simulink model "c00002M_harness"  (R2018a)
settings: Solver=FixedStepAuto  StartTime=0.0  StopTime=300  FixedStep=0.1  RelTol=1e-3
undefined symbols (not defined in the file): A1, hmax, R1, R2, sigbuilder_block, TempThreshold
(part 1 of 14)
settings Model: Creator=aarrieta  LastModifiedBy=umarkiegi

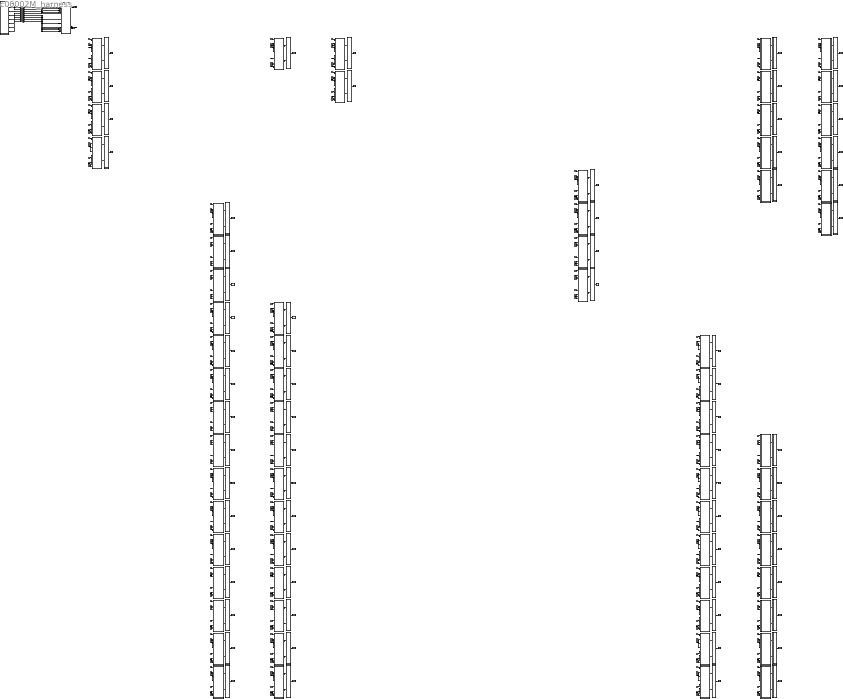
== system c00002M_harness ==
  CPSUT : Subsystem
  Eval : Subsystem
  Eval1 : Subsystem
  Eval164 : Subsystem
  Eval165 : Subsystem
  Eval166 : Subsystem
  Eval167 : Subsystem
  Eval2 : Subsystem
  Eval209 : Subsystem
  Eval210 : Subsystem
  Eval211 : Subsystem
  Eval212 : Subsystem
  Eval213 : Subsystem
  Eval214 : Subsystem
  Eval215 : Subsystem
  Eval216 : Subsystem
  Eval217 : Subsystem
  Eval218 : Subsystem
  Eval219 : Subsystem
  Eval220 : Subsystem
  Eval221 : Subsystem
  Eval222 : Subsystem
  Eval223 : Subsystem
  Eval224 : Subsystem
  Eval232 : Subsystem
  Eval233 : Subsystem
  Eval234 : Subsystem
  Eval235 : Subsystem
  Eval236 : Subsystem
  Eval237 : Subsystem
  Eval238 : Subsystem
  Eval239 : Subsystem
  Eval240 : Subsystem
  Eval241 : Subsystem
  Eval242 : Subsystem
  Eval243 : Subsystem
  Eval244 : Subsystem
  Eval245 : Subsystem
  Eval3 : Subsystem
  Eval45 : Subsystem
  Eval46 : Subsystem
  Eval47 : Subsystem
  Eval48 : Subsystem
  Eval49 : Subsystem
  Eval50 : Subsystem
  Eval51 : Subsystem
  Eval52 : Subsystem
  Eval53 : Subsystem
  Eval54 : Subsystem
  Eval55 : Subsystem
  Eval56 : Subsystem
  Eval57 : Subsystem
  Eval58 : Subsystem
  Eval59 : Subsystem
  Eval60 : Subsystem
  Eval68 : Subsystem
  Eval69 : Subsystem
  Eval70 : Subsystem
  Eval71 : Subsystem
  Eval72 : Subsystem
  Eval73 : Subsystem
  Eval74 : Subsystem
  Eval75 : Subsystem
  Eval76 : Subsystem
  Eval77 : Subsystem
  Eval78 : Subsystem
  Eval79 : Subsystem
  Eval80 : Subsystem
  Eval81 : Subsystem
  Inputs : Subsystem  Tag=STV Subsys  LoadFcn=sigbuilder_block('load');  StartFcn=sigbuilder_block('start');  StopFcn=sigbuilder_block('stop');  ClipboardFcn=sigbuilder_block('clipboard');  mask(Sigbuilder block){tuvar=[0:10]}
      mask init:
      | if ~strcmp(get_param(bdroot(gcb),'SimulationStatus'),'stopped'),tuvar = sigbuilder_block('maskInit'); end
      settings: CopyFcn=sigbuilder_block('copy');  DeleteFcn=sigbuilder_block('delete');  ModelCloseFcn=sigbuilder_block('modelClose');  PreSaveFcn=sigbuilder_block('preSave');  PauseFcn=sigbuilder_block('pause');  ContinueFcn=sigbuilder_block('continue');  NameChangeFcn=sigbuilder_block('namechange');  OpenFcn=sigbuilder_block('open',[276.75 163.5 675.75 486.75 ]);  CloseFcn=sigbuilder_block('close');
      mask Display: plot(0, 0, 100, 100,[2, 2, 32, 32, 2], [68, 8, 8, 68, 68],[32, 2], [38, 38], [32, 19, 2],[53, 60, 44], [32, 17, 17, 2],[16, 16, 31, 31]);txt = getActiveGroup(gcbh);text(2, 100, txt,'verticalAlignment', 'top');
  M001 : Subsystem
  M002 : Subsystem
  M003 : Subsystem
  M004 : Subsystem
  M046 : Subsystem
  M047 : Subsystem
  M048 : Subsystem
  M049 : Subsystem
  M050 : Subsystem
  M051 : Subsystem
  M052 : Subsystem
  M053 : Subsystem
  M054 : Subsystem
  M055 : Subsystem
  M056 : Subsystem
  M057 : Subsystem
  M058 : Subsystem
  M059 : Subsystem
  M060 : Subsystem
  M061 : Subsystem
  M069 : Subsystem
  M070 : Subsystem
  M071 : Subsystem
  M072 : Subsystem
  M073 : Subsystem
  M074 : Subsystem
  M075 : Subsystem
  M076 : Subsystem
  M077 : Subsystem
  M078 : Subsystem
  M079 : Subsystem
  M080 : Subsystem
  M081 : Subsystem
  M082 : Subsystem
  M165 : Subsystem
  M166 : Subsystem
  M167 : Subsystem
  M168 : Subsystem
  M210 : Subsystem
  M211 : Subsystem
  M212 : Subsystem
  M213 : Subsystem
  M214 : Subsystem
  M215 : Subsystem
  M216 : Subsystem
  M217 : Subsystem
  M218 : Subsystem
  M219 : Subsystem
  M220 : Subsystem
  M221 : Subsystem
  M222 : Subsystem
  M223 : Subsystem
  M224 : Subsystem
  M225 : Subsystem
  M233 : Subsystem
  M234 : Subsystem
  M235 : Subsystem
  M236 : Subsystem
  M237 : Subsystem
  M238 : Subsystem
  M239 : Subsystem
  M240 : Subsystem
  M241 : Subsystem
  M242 : Subsystem
  M243 : Subsystem
  M244 : Subsystem
  M245 : Subsystem
  M246 : Subsystem
  To Workspace : ToWorkspace  VariableName=mutant001  SampleTime=-1
  To Workspace1 : ToWorkspace  VariableName=mutant002  SampleTime=-1
  To Workspace164 : ToWorkspace  VariableName=mutant165  SampleTime=-1
  To Workspace165 : ToWorkspace  VariableName=mutant166  SampleTime=-1
  To Workspace166 : ToWorkspace  VariableName=mutant167  SampleTime=-1
  To Workspace167 : ToWorkspace  VariableName=mutant168  SampleTime=-1
  To Workspace2 : ToWorkspace  VariableName=mutant003  SampleTime=-1
  To Workspace209 : ToWorkspace  VariableName=mutant210  SampleTime=-1
  To Workspace210 : ToWorkspace  VariableName=mutant211  SampleTime=-1
  To Workspace211 : ToWorkspace  VariableName=mutant212  SampleTime=-1
  To Workspace212 : ToWorkspace  VariableName=mutant213  SampleTime=-1
  To Workspace213 : ToWorkspace  VariableName=mutant214  SampleTime=-1
  To Workspace214 : ToWorkspace  VariableName=mutant215  SampleTime=-1
  To Workspace215 : ToWorkspace  VariableName=mutant216  SampleTime=-1
  To Workspace216 : ToWorkspace  VariableName=mutant217  SampleTime=-1
  To Workspace217 : ToWorkspace  VariableName=mutant218  SampleTime=-1
  To Workspace218 : ToWorkspace  VariableName=mutant219  SampleTime=-1
  To Workspace219 : ToWorkspace  VariableName=mutant220  SampleTime=-1
  To Workspace220 : ToWorkspace  VariableName=mutant221  SampleTime=-1
  To Workspace221 : ToWorkspace  VariableName=mutant222  SampleTime=-1
  To Workspace222 : ToWorkspace  VariableName=mutant223  SampleTime=-1
  To Workspace223 : ToWorkspace  VariableName=mutant224  SampleTime=-1
  To Workspace224 : ToWorkspace  VariableName=mutant225  SampleTime=-1
  To Workspace232 : ToWorkspace  VariableName=mutant233  SampleTime=-1
  To Workspace233 : ToWorkspace  VariableName=mutant234  SampleTime=-1
  To Workspace234 : ToWorkspace  VariableName=mutant235  SampleTime=-1
  To Workspace235 : ToWorkspace  VariableName=mutant236  SampleTime=-1
  To Workspace236 : ToWorkspace  VariableName=mutant237  SampleTime=-1
  To Workspace237 : ToWorkspace  VariableName=mutant238  SampleTime=-1
  To Workspace238 : ToWorkspace  VariableName=mutant239  SampleTime=-1
  To Workspace239 : ToWorkspace  VariableName=mutant240  SampleTime=-1
  To Workspace240 : ToWorkspace  VariableName=mutant241  SampleTime=-1
  To Workspace241 : ToWorkspace  VariableName=mutant242  SampleTime=-1
  To Workspace242 : ToWorkspace  VariableName=mutant243  SampleTime=-1
  To Workspace243 : ToWorkspace  VariableName=mutant244  SampleTime=-1
  To Workspace244 : ToWorkspace  VariableName=mutant245  SampleTime=-1
  To Workspace245 : ToWorkspace  VariableName=mutant246  SampleTime=-1
  To Workspace3 : ToWorkspace  VariableName=mutant004  SampleTime=-1
  To Workspace45 : ToWorkspace  VariableName=mutant046  SampleTime=-1
  To Workspace46 : ToWorkspace  VariableName=mutant047  SampleTime=-1
  To Workspace47 : ToWorkspace  VariableName=mutant048  SampleTime=-1
  To Workspace48 : ToWorkspace  VariableName=mutant049  SampleTime=-1
  To Workspace49 : ToWorkspace  VariableName=mutant050  SampleTime=-1
  To Workspace50 : ToWorkspace  VariableName=mutant051  SampleTime=-1
  To Workspace51 : ToWorkspace  VariableName=mutant052  SampleTime=-1
  To Workspace52 : ToWorkspace  VariableName=mutant053  SampleTime=-1
  To Workspace53 : ToWorkspace  VariableName=mutant054  SampleTime=-1
  To Workspace54 : ToWorkspace  VariableName=mutant055  SampleTime=-1
  To Workspace55 : ToWorkspace  VariableName=mutant056  SampleTime=-1
  To Workspace56 : ToWorkspace  VariableName=mutant057  SampleTime=-1
  To Workspace57 : ToWorkspace  VariableName=mutant058  SampleTime=-1
  To Workspace58 : ToWorkspace  VariableName=mutant059  SampleTime=-1
  To Workspace59 : ToWorkspace  VariableName=mutant060  SampleTime=-1
  To Workspace60 : ToWorkspace  VariableName=mutant061  SampleTime=-1
  To Workspace68 : ToWorkspace  VariableName=mutant069  SampleTime=-1
  To Workspace69 : ToWorkspace  VariableName=mutant070  SampleTime=-1
  To Workspace70 : ToWorkspace  VariableName=mutant071  SampleTime=-1
  To Workspace71 : ToWorkspace  VariableName=mutant072  SampleTime=-1
  To Workspace72 : ToWorkspace  VariableName=mutant073  SampleTime=-1
  To Workspace73 : ToWorkspace  VariableName=mutant074  SampleTime=-1
  To Workspace74 : ToWorkspace  VariableName=mutant075  SampleTime=-1
  To Workspace75 : ToWorkspace  VariableName=mutant076  SampleTime=-1
  To Workspace76 : ToWorkspace  VariableName=mutant077  SampleTime=-1
  To Workspace77 : ToWorkspace  VariableName=mutant078  SampleTime=-1
  To Workspace78 : ToWorkspace  VariableName=mutant079  SampleTime=-1
  To Workspace79 : ToWorkspace  VariableName=mutant080  SampleTime=-1
  To Workspace80 : ToWorkspace  VariableName=mutant081  SampleTime=-1
  To Workspace81 : ToWorkspace  VariableName=mutant082  SampleTime=-1
  dtc_CT1 : DataTypeConversion
  dtc_CT3 : DataTypeConversion
  dtc_EB1 : DataTypeConversion
  dtc_EB3 : DataTypeConversion
  dtc_MR1 : DataTypeConversion
  dtc_MR3 : DataTypeConversion
  dtc_T1 : DataTypeConversion
  dtc_T3 : DataTypeConversion
  LL1 : Outport
  LL3 : Outport  Port=2
  tag scope: out1=global, out3=global
  wires:
  CPSUT/1(LL1) -> [out1], LL1/1
  CPSUT/2(LL3) -> [out3], LL3/1
  [in1] -> M001/1(CT1)
  [in4] -> M001/2(MR1)
  [in5] -> M001/3(T1)
  [in6] -> M001/4(EB1)
  [in13] -> M001/5(CT3)
  [in16] -> M001/6(MR3)
  [in17] -> M001/7(T3)
  [in18] -> M001/8(EB3)
  Eval/1(Out1) -> To Workspace/1
  M001/1(LL1) -> Eval/1(In1)
  M001/2(LL3) -> Eval/2(In3)
  [in1] -> M002/1(CT1)
  [in4] -> M002/2(MR1)
  [in5] -> M002/3(T1)
  [in6] -> M002/4(EB1)
  [in13] -> M002/5(CT3)
  [in16] -> M002/6(MR3)
  [in17] -> M002/7(T3)
  [in18] -> M002/8(EB3)
  M002/1(LL1) -> Eval1/1(In1)
  M002/2(LL3) -> Eval1/2(In3)
  Eval1/1(Out1) -> To Workspace1/1
  [in1] -> M003/1(CT1)
  [in4] -> M003/2(MR1)
  [in5] -> M003/3(T1)
  [in6] -> M003/4(EB1)
  [in13] -> M003/5(CT3)
  [in16] -> M003/6(MR3)
  [in17] -> M003/7(T3)
  [in18] -> M003/8(EB3)
  M003/1(LL1) -> Eval2/1(In1)
  M003/2(LL3) -> Eval2/2(In3)
  Eval2/1(Out1) -> To Workspace2/1
  [in1] -> M004/1(CT1)
  [in4] -> M004/2(MR1)
  [in5] -> M004/3(T1)
  [in6] -> M004/4(EB1)
  [in13] -> M004/5(CT3)
  [in16] -> M004/6(MR3)
  [in17] -> M004/7(T3)
  [in18] -> M004/8(EB3)
  M004/1(LL1) -> Eval3/1(In1)
  M004/2(LL3) -> Eval3/2(In3)
  Eval3/1(Out1) -> To Workspace3/1
  [in1] -> M046/1(CT1)
  [in4] -> M046/2(MR1)
  [in5] -> M046/3(T1)
  [in6] -> M046/4(EB1)
  [in13] -> M046/5(CT3)
  [in16] -> M046/6(MR3)
  [in17] -> M046/7(T3)
  [in18] -> M046/8(EB3)
  M046/1(LL1) -> Eval45/1(In1)
  M046/2(LL3) -> Eval45/2(In3)
  Eval45/1(Out1) -> To Workspace45/1
  [in1] -> M047/1(CT1)
  [in4] -> M047/2(MR1)
  [in5] -> M047/3(T1)
  [in6] -> M047/4(EB1)
  [in13] -> M047/5(CT3)
  [in16] -> M047/6(MR3)
  [in17] -> M047/7(T3)
  [in18] -> M047/8(EB3)
  M047/1(LL1) -> Eval46/1(In1)
  M047/2(LL3) -> Eval46/2(In3)
  Eval46/1(Out1) -> To Workspace46/1
  [in1] -> M048/1(CT1)
  [in4] -> M048/2(MR1)
  [in5] -> M048/3(T1)
  [in6] -> M048/4(EB1)
  [in13] -> M048/5(CT3)
  [in16] -> M048/6(MR3)
  [in17] -> M048/7(T3)
  [in18] -> M048/8(EB3)
  M048/1(LL1) -> Eval47/1(In1)
  M048/2(LL3) -> Eval47/2(In3)
  Eval47/1(Out1) -> To Workspace47/1
  [in1] -> M049/1(CT1)
  [in4] -> M049/2(MR1)
  [in5] -> M049/3(T1)
  [in6] -> M049/4(EB1)
  [in13] -> M049/5(CT3)
  [in16] -> M049/6(MR3)
  [in17] -> M049/7(T3)
  [in18] -> M049/8(EB3)
  M049/1(LL1) -> Eval48/1(In1)
  M049/2(LL3) -> Eval48/2(In3)
  Eval48/1(Out1) -> To Workspace48/1
  [in1] -> M050/1(CT1)
  [in4] -> M050/2(MR1)
  [in5] -> M050/3(T1)
  [in6] -> M050/4(EB1)
  [in13] -> M050/5(CT3)
  [in16] -> M050/6(MR3)
  [in17] -> M050/7(T3)
  [in18] -> M050/8(EB3)
  M050/1(LL1) -> Eval49/1(In1)
  M050/2(LL3) -> Eval49/2(In3)
  Eval49/1(Out1) -> To Workspace49/1
  [in1] -> M051/1(CT1)
  [in4] -> M051/2(MR1)
  [in5] -> M051/3(T1)
  [in6] -> M051/4(EB1)
  [in13] -> M051/5(CT3)
  [in16] -> M051/6(MR3)
  [in17] -> M051/7(T3)
  [in18] -> M051/8(EB3)
  M051/1(LL1) -> Eval50/1(In1)
  M051/2(LL3) -> Eval50/2(In3)
  Eval50/1(Out1) -> To Workspace50/1
  [in1] -> M052/1(CT1)
  [in4] -> M052/2(MR1)
  [in5] -> M052/3(T1)
  [in6] -> M052/4(EB1)
  [in13] -> M052/5(CT3)
  [in16] -> M052/6(MR3)
  [in17] -> M052/7(T3)
  [in18] -> M052/8(EB3)
  M052/1(LL1) -> Eval51/1(In1)
  M052/2(LL3) -> Eval51/2(In3)
  Eval51/1(Out1) -> To Workspace51/1
  [in1] -> M053/1(CT1)
  [in4] -> M053/2(MR1)
  [in5] -> M053/3(T1)
  [in6] -> M053/4(EB1)
  [in13] -> M053/5(CT3)
  [in16] -> M053/6(MR3)
  [in17] -> M053/7(T3)
  [in18] -> M053/8(EB3)
  M053/1(LL1) -> Eval52/1(In1)
  M053/2(LL3) -> Eval52/2(In3)
  Eval52/1(Out1) -> To Workspace52/1
  [in1] -> M054/1(CT1)
  [in4] -> M054/2(MR1)
  [in5] -> M054/3(T1)
  [in6] -> M054/4(EB1)
  [in13] -> M054/5(CT3)
  [in16] -> M054/6(MR3)
  [in17] -> M054/7(T3)
  [in18] -> M054/8(EB3)
  M054/1(LL1) -> Eval53/1(In1)
  M054/2(LL3) -> Eval53/2(In3)
  Eval53/1(Out1) -> To Workspace53/1
  [in1] -> M055/1(CT1)
  [in4] -> M055/2(MR1)
  [in5] -> M055/3(T1)
  [in6] -> M055/4(EB1)
  [in13] -> M055/5(CT3)
  [in16] -> M055/6(MR3)
  [in17] -> M055/7(T3)
  [in18] -> M055/8(EB3)
  M055/1(LL1) -> Eval54/1(In1)
  M055/2(LL3) -> Eval54/2(In3)
  Eval54/1(Out1) -> To Workspace54/1
  [in1] -> M056/1(CT1)
  [in4] -> M056/2(MR1)
  [in5] -> M056/3(T1)
  [in6] -> M056/4(EB1)
  [in13] -> M056/5(CT3)
  [in16] -> M056/6(MR3)
  [in17] -> M056/7(T3)
  [in18] -> M056/8(EB3)
  M056/1(LL1) -> Eval55/1(In1)
  M056/2(LL3) -> Eval55/2(In3)
  Eval55/1(Out1) -> To Workspace55/1
  [in1] -> M057/1(CT1)
  [in4] -> M057/2(MR1)
  [in5] -> M057/3(T1)
  [in6] -> M057/4(EB1)
  [in13] -> M057/5(CT3)
  [in16] -> M057/6(MR3)
  [in17] -> M057/7(T3)
  [in18] -> M057/8(EB3)
  M057/1(LL1) -> Eval56/1(In1)
  M057/2(LL3) -> Eval56/2(In3)
  Eval56/1(Out1) -> To Workspace56/1
  [in1] -> M058/1(CT1)
  [in4] -> M058/2(MR1)
  [in5] -> M058/3(T1)
  [in6] -> M058/4(EB1)
  [in13] -> M058/5(CT3)
  [in16] -> M058/6(MR3)
  [in17] -> M058/7(T3)
  [in18] -> M058/8(EB3)
  M058/1(LL1) -> Eval57/1(In1)
  M058/2(LL3) -> Eval57/2(In3)
  Eval57/1(Out1) -> To Workspace57/1
  [in1] -> M059/1(CT1)
  [in4] -> M059/2(MR1)
  [in5] -> M059/3(T1)
  [in6] -> M059/4(EB1)
  [in13] -> M059/5(CT3)
  [in16] -> M059/6(MR3)
  [in17] -> M059/7(T3)
  [in18] -> M059/8(EB3)
  M059/1(LL1) -> Eval58/1(In1)
  M059/2(LL3) -> Eval58/2(In3)
  Eval58/1(Out1) -> To Workspace58/1
  [in1] -> M060/1(CT1)
  [in4] -> M060/2(MR1)
  [in5] -> M060/3(T1)
  [in6] -> M060/4(EB1)
  [in13] -> M060/5(CT3)
  [in16] -> M060/6(MR3)
  [in17] -> M060/7(T3)
  [in18] -> M060/8(EB3)
  M060/1(LL1) -> Eval59/1(In1)
  M060/2(LL3) -> Eval59/2(In3)
  Eval59/1(Out1) -> To Workspace59/1
  [in1] -> M061/1(CT1)
  [in4] -> M061/2(MR1)
  [in5] -> M061/3(T1)
  [in6] -> M061/4(EB1)
  [in13] -> M061/5(CT3)
  [in16] -> M061/6(MR3)
  [in17] -> M061/7(T3)
  [in18] -> M061/8(EB3)
  M061/1(LL1) -> Eval60/1(In1)
  M061/2(LL3) -> Eval60/2(In3)
  Eval60/1(Out1) -> To Workspace60/1
  [in1] -> M069/1(CT1)
  [in4] -> M069/2(MR1)
  [in5] -> M069/3(T1)
  [in6] -> M069/4(EB1)
  [in13] -> M069/5(CT3)
  [in16] -> M069/6(MR3)
  [in17] -> M069/7(T3)
  [in18] -> M069/8(EB3)
  M069/1(LL1) -> Eval68/1(In1)
  M069/2(LL3) -> Eval68/2(In3)
  Eval68/1(Out1) -> To Workspace68/1
  [in1] -> M070/1(CT1)
  [in4] -> M070/2(MR1)
  [in5] -> M070/3(T1)
  [in6] -> M070/4(EB1)
  [in13] -> M070/5(CT3)
  [in16] -> M070/6(MR3)
  [in17] -> M070/7(T3)
  [in18] -> M070/8(EB3)
  M070/1(LL1) -> Eval69/1(In1)
  M070/2(LL3) -> Eval69/2(In3)
  Eval69/1(Out1) -> To Workspace69/1
  [in1] -> M071/1(CT1)
  [in4] -> M071/2(MR1)
  [in5] -> M071/3(T1)
  [in6] -> M071/4(EB1)
  [in13] -> M071/5(CT3)
  [in16] -> M071/6(MR3)
  [in17] -> M071/7(T3)
  [in18] -> M071/8(EB3)
  M071/1(LL1) -> Eval70/1(In1)
  M071/2(LL3) -> Eval70/2(In3)
  Eval70/1(Out1) -> To Workspace70/1
  [in1] -> M072/1(CT1)
  [in4] -> M072/2(MR1)
  [in5] -> M072/3(T1)
  [in6] -> M072/4(EB1)
  [in13] -> M072/5(CT3)
  [in16] -> M072/6(MR3)
  [in17] -> M072/7(T3)
  [in18] -> M072/8(EB3)
  M072/1(LL1) -> Eval71/1(In1)
  M072/2(LL3) -> Eval71/2(In3)
  Eval71/1(Out1) -> To Workspace71/1
  [in1] -> M073/1(CT1)
  [in4] -> M073/2(MR1)
  [in5] -> M073/3(T1)
  [in6] -> M073/4(EB1)
  [in13] -> M073/5(CT3)
  [in16] -> M073/6(MR3)
  [in17] -> M073/7(T3)
  [in18] -> M073/8(EB3)
  M073/1(LL1) -> Eval72/1(In1)
  M073/2(LL3) -> Eval72/2(In3)
  Eval72/1(Out1) -> To Workspace72/1
  [in1] -> M074/1(CT1)
  [in4] -> M074/2(MR1)
  [in5] -> M074/3(T1)
  [in6] -> M074/4(EB1)
  [in13] -> M074/5(CT3)
  [in16] -> M074/6(MR3)
  [in17] -> M074/7(T3)
  [in18] -> M074/8(EB3)
  M074/1(LL1) -> Eval73/1(In1)
  M074/2(LL3) -> Eval73/2(In3)
  Eval73/1(Out1) -> To Workspace73/1
  [in1] -> M075/1(CT1)
  [in4] -> M075/2(MR1)
  [in5] -> M075/3(T1)
  [in6] -> M075/4(EB1)
  [in13] -> M075/5(CT3)
  [in16] -> M075/6(MR3)
  [in17] -> M075/7(T3)
  [in18] -> M075/8(EB3)
  M075/1(LL1) -> Eval74/1(In1)
  M075/2(LL3) -> Eval74/2(In3)
  Eval74/1(Out1) -> To Workspace74/1
  [in1] -> M076/1(CT1)
  [in4] -> M076/2(MR1)
  [in5] -> M076/3(T1)
  [in6] -> M076/4(EB1)
  [in13] -> M076/5(CT3)
  [in16] -> M076/6(MR3)
  [in17] -> M076/7(T3)
  [in18] -> M076/8(EB3)
  M076/1(LL1) -> Eval75/1(In1)
  M076/2(LL3) -> Eval75/2(In3)
  Eval75/1(Out1) -> To Workspace75/1
  [in1] -> M077/1(CT1)
  [in4] -> M077/2(MR1)
  [in5] -> M077/3(T1)
  [in6] -> M077/4(EB1)
  [in13] -> M077/5(CT3)
  [in16] -> M077/6(MR3)
  [in17] -> M077/7(T3)
  [in18] -> M077/8(EB3)
  M077/1(LL1) -> Eval76/1(In1)
  M077/2(LL3) -> Eval76/2(In3)
  Eval76/1(Out1) -> To Workspace76/1
  [in1] -> M078/1(CT1)
  [in4] -> M078/2(MR1)
  [in5] -> M078/3(T1)
  [in6] -> M078/4(EB1)
  [in13] -> M078/5(CT3)
  [in16] -> M078/6(MR3)
  [in17] -> M078/7(T3)
  [in18] -> M078/8(EB3)
  M078/1(LL1) -> Eval77/1(In1)
  M078/2(LL3) -> Eval77/2(In3)
  Eval77/1(Out1) -> To Workspace77/1
  [in1] -> M079/1(CT1)
  [in4] -> M079/2(MR1)
  [in5] -> M079/3(T1)
  [in6] -> M079/4(EB1)
  [in13] -> M079/5(CT3)
  [in16] -> M079/6(MR3)
  [in17] -> M079/7(T3)
  [in18] -> M079/8(EB3)
  M079/1(LL1) -> Eval78/1(In1)
  M079/2(LL3) -> Eval78/2(In3)
  Eval78/1(Out1) -> To Workspace78/1
  [in1] -> M080/1(CT1)
  [in4] -> M080/2(MR1)
  [in5] -> M080/3(T1)
  [in6] -> M080/4(EB1)
  [in13] -> M080/5(CT3)
  [in16] -> M080/6(MR3)
  [in17] -> M080/7(T3)
  [in18] -> M080/8(EB3)
  M080/1(LL1) -> Eval79/1(In1)
  M080/2(LL3) -> Eval79/2(In3)
  Eval79/1(Out1) -> To Workspace79/1
  [in1] -> M081/1(CT1)
  [in4] -> M081/2(MR1)
  [in5] -> M081/3(T1)
  [in6] -> M081/4(EB1)
  [in13] -> M081/5(CT3)
  [in16] -> M081/6(MR3)
  [in17] -> M081/7(T3)
  [in18] -> M081/8(EB3)
  M081/1(LL1) -> Eval80/1(In1)
  M081/2(LL3) -> Eval80/2(In3)
  Eval80/1(Out1) -> To Workspace80/1
  [in1] -> M082/1(CT1)
  [in4] -> M082/2(MR1)
  [in5] -> M082/3(T1)
  [in6] -> M082/4(EB1)
  [in13] -> M082/5(CT3)
  [in16] -> M082/6(MR3)
  [in17] -> M082/7(T3)
  [in18] -> M082/8(EB3)
  M082/1(LL1) -> Eval81/1(In1)
  M082/2(LL3) -> Eval81/2(In3)
  Eval81/1(Out1) -> To Workspace81/1
  [in1] -> M165/1(CT1)
  [in4] -> M165/2(MR1)
  [in5] -> M165/3(T1)
  [in6] -> M165/4(EB1)
  [in13] -> M165/5(CT3)
  [in16] -> M165/6(MR3)
  [in17] -> M165/7(T3)
  [in18] -> M165/8(EB3)
  M165/1(LL1) -> Eval164/1(In1)
  M165/2(LL3) -> Eval164/2(In3)
  Eval164/1(Out1) -> To Workspace164/1
  [in1] -> M166/1(CT1)
  [in4] -> M166/2(MR1)
  [in5] -> M166/3(T1)
  [in6] -> M166/4(EB1)
  [in13] -> M166/5(CT3)
  [in16] -> M166/6(MR3)
  [in17] -> M166/7(T3)
  [in18] -> M166/8(EB3)
  M166/1(LL1) -> Eval165/1(In1)
  M166/2(LL3) -> Eval165/2(In3)
  Eval165/1(Out1) -> To Workspace165/1
  [in1] -> M167/1(CT1)
  [in4] -> M167/2(MR1)
  [in5] -> M167/3(T1)
  [in6] -> M167/4(EB1)
  [in13] -> M167/5(CT3)
  [in16] -> M167/6(MR3)
  [in17] -> M167/7(T3)
  [in18] -> M167/8(EB3)
  M167/1(LL1) -> Eval166/1(In1)
  M167/2(LL3) -> Eval166/2(In3)
  Eval166/1(Out1) -> To Workspace166/1
  [in1] -> M168/1(CT1)
  [in4] -> M168/2(MR1)
  [in5] -> M168/3(T1)
  [in6] -> M168/4(EB1)
  [in13] -> M168/5(CT3)
  [in16] -> M168/6(MR3)
  [in17] -> M168/7(T3)
  [in18] -> M168/8(EB3)
  M168/1(LL1) -> Eval167/1(In1)
  M168/2(LL3) -> Eval167/2(In3)
  Eval167/1(Out1) -> To Workspace167/1
  [in1] -> M210/1(CT1)
  [in4] -> M210/2(MR1)
  [in5] -> M210/3(T1)
  [in6] -> M210/4(EB1)
  [in13] -> M210/5(CT3)
  [in16] -> M210/6(MR3)
  [in17] -> M210/7(T3)
  [in18] -> M210/8(EB3)
  M210/1(LL1) -> Eval209/1(In1)
  M210/2(LL3) -> Eval209/2(In3)
  Eval209/1(Out1) -> To Workspace209/1
  [in1] -> M211/1(CT1)
  [in4] -> M211/2(MR1)
  [in5] -> M211/3(T1)
  [in6] -> M211/4(EB1)
  [in13] -> M211/5(CT3)
  [in16] -> M211/6(MR3)
  [in17] -> M211/7(T3)
  [in18] -> M211/8(EB3)
  M211/1(LL1) -> Eval210/1(In1)
  M211/2(LL3) -> Eval210/2(In3)
  Eval210/1(Out1) -> To Workspace210/1
  [in1] -> M212/1(CT1)
  [in4] -> M212/2(MR1)
  [in5] -> M212/3(T1)
  [in6] -> M212/4(EB1)
  [in13] -> M212/5(CT3)
  [in16] -> M212/6(MR3)
  [in17] -> M212/7(T3)
  [in18] -> M212/8(EB3)
  M212/1(LL1) -> Eval211/1(In1)
  M212/2(LL3) -> Eval211/2(In3)
  Eval211/1(Out1) -> To Workspace211/1
  [in1] -> M213/1(CT1)
  [in4] -> M213/2(MR1)
  [in5] -> M213/3(T1)
  [in6] -> M213/4(EB1)
  [in13] -> M213/5(CT3)
  [in16] -> M213/6(MR3)
  [in17] -> M213/7(T3)
  [in18] -> M213/8(EB3)
  M213/1(LL1) -> Eval212/1(In1)
  M213/2(LL3) -> Eval212/2(In3)
  Eval212/1(Out1) -> To Workspace212/1
  [in1] -> M214/1(CT1)
  [in4] -> M214/2(MR1)
  [in5] -> M214/3(T1)
  [in6] -> M214/4(EB1)
  [in13] -> M214/5(CT3)
  [in16] -> M214/6(MR3)
  [in17] -> M214/7(T3)
  [in18] -> M214/8(EB3)
  M214/1(LL1) -> Eval213/1(In1)
  M214/2(LL3) -> Eval213/2(In3)
  Eval213/1(Out1) -> To Workspace213/1
  [in1] -> M215/1(CT1)
  [in4] -> M215/2(MR1)
  [in5] -> M215/3(T1)
  [in6] -> M215/4(EB1)
  [in13] -> M215/5(CT3)
  [in16] -> M215/6(MR3)
  [in17] -> M215/7(T3)
  [in18] -> M215/8(EB3)
  M215/1(LL1) -> Eval214/1(In1)
  M215/2(LL3) -> Eval214/2(In3)
  Eval214/1(Out1) -> To Workspace214/1
  [in1] -> M216/1(CT1)
  [in4] -> M216/2(MR1)
  [in5] -> M216/3(T1)
  [in6] -> M216/4(EB1)
  [in13] -> M216/5(CT3)
  [in16] -> M216/6(MR3)
  [in17] -> M216/7(T3)
  [in18] -> M216/8(EB3)
  M216/1(LL1) -> Eval215/1(In1)
  M216/2(LL3) -> Eval215/2(In3)
  Eval215/1(Out1) -> To Workspace215/1
  [in1] -> M217/1(CT1)
  [in4] -> M217/2(MR1)
  [in5] -> M217/3(T1)
  [in6] -> M217/4(EB1)
  [in13] -> M217/5(CT3)
  [in16] -> M217/6(MR3)
  [in17] -> M217/7(T3)
  [in18] -> M217/8(EB3)
  M217/1(LL1) -> Eval216/1(In1)
  M217/2(LL3) -> Eval216/2(In3)
  Eval216/1(Out1) -> To Workspace216/1
  [in1] -> M218/1(CT1)
  [in4] -> M218/2(MR1)
  [in5] -> M218/3(T1)
  [in6] -> M218/4(EB1)
  [in13] -> M218/5(CT3)
  [in16] -> M218/6(MR3)
  [in17] -> M218/7(T3)
  [in18] -> M218/8(EB3)
  M218/1(LL1) -> Eval217/1(In1)
  M218/2(LL3) -> Eval217/2(In3)
  Eval217/1(Out1) -> To Workspace217/1
  [in1] -> M219/1(CT1)
  [in4] -> M219/2(MR1)
  [in5] -> M219/3(T1)
  [in6] -> M219/4(EB1)
  [in13] -> M219/5(CT3)
  [in16] -> M219/6(MR3)
  [in17] -> M219/7(T3)
  [in18] -> M219/8(EB3)
  M219/1(LL1) -> Eval218/1(In1)
  M219/2(LL3) -> Eval218/2(In3)
  Eval218/1(Out1) -> To Workspace218/1
  [in1] -> M220/1(CT1)
  [in4] -> M220/2(MR1)
  [in5] -> M220/3(T1)
  [in6] -> M220/4(EB1)
  [in13] -> M220/5(CT3)
  [in16] -> M220/6(MR3)
  [in17] -> M220/7(T3)
  [in18] -> M220/8(EB3)
  M220/1(LL1) -> Eval219/1(In1)
  M220/2(LL3) -> Eval219/2(In3)
  Eval219/1(Out1) -> To Workspace219/1
  [in1] -> M221/1(CT1)
  [in4] -> M221/2(MR1)
  [in5] -> M221/3(T1)
  [in6] -> M221/4(EB1)
  [in13] -> M221/5(CT3)
  [in16] -> M221/6(MR3)
  [in17] -> M221/7(T3)
  [in18] -> M221/8(EB3)
  M221/1(LL1) -> Eval220/1(In1)
  M221/2(LL3) -> Eval220/2(In3)
  Eval220/1(Out1) -> To Workspace220/1
  [in1] -> M222/1(CT1)
  [in4] -> M222/2(MR1)
  [in5] -> M222/3(T1)
  [in6] -> M222/4(EB1)
  [in13] -> M222/5(CT3)
  [in16] -> M222/6(MR3)
  [in17] -> M222/7(T3)
  [in18] -> M222/8(EB3)
  M222/1(LL1) -> Eval221/1(In1)
  M222/2(LL3) -> Eval221/2(In3)
  Eval221/1(Out1) -> To Workspace221/1
  [in1] -> M223/1(CT1)
  [in4] -> M223/2(MR1)
  [in5] -> M223/3(T1)
  [in6] -> M223/4(EB1)
  [in13] -> M223/5(CT3)
  [in16] -> M223/6(MR3)
  [in17] -> M223/7(T3)
  [in18] -> M223/8(EB3)
  M223/1(LL1) -> Eval222/1(In1)
  M223/2(LL3) -> Eval222/2(In3)
  Eval222/1(Out1) -> To Workspace222/1
  [in1] -> M224/1(CT1)
  [in4] -> M224/2(MR1)
  [in5] -> M224/3(T1)
  [in6] -> M224/4(EB1)
  [in13] -> M224/5(CT3)
  [in16] -> M224/6(MR3)
  [in17] -> M224/7(T3)
  [in18] -> M224/8(EB3)
  M224/1(LL1) -> Eval223/1(In1)
  M224/2(LL3) -> Eval223/2(In3)
  Eval223/1(Out1) -> To Workspace223/1
  [in1] -> M225/1(CT1)
  [in4] -> M225/2(MR1)
  [in5] -> M225/3(T1)
  [in6] -> M225/4(EB1)
  [in13] -> M225/5(CT3)
  [in16] -> M225/6(MR3)
  [in17] -> M225/7(T3)
  [in18] -> M225/8(EB3)
  M225/1(LL1) -> Eval224/1(In1)
  M225/2(LL3) -> Eval224/2(In3)
  Eval224/1(Out1) -> To Workspace224/1
  [in1] -> M233/1(CT1)
  [in4] -> M233/2(MR1)
  [in5] -> M233/3(T1)
  [in6] -> M233/4(EB1)
  [in13] -> M233/5(CT3)
  [in16] -> M233/6(MR3)
  [in17] -> M233/7(T3)
  [in18] -> M233/8(EB3)
  M233/1(LL1) -> Eval232/1(In1)
  M233/2(LL3) -> Eval232/2(In3)
  Eval232/1(Out1) -> To Workspace232/1
  [in1] -> M234/1(CT1)
  [in4] -> M234/2(MR1)
  [in5] -> M234/3(T1)
  [in6] -> M234/4(EB1)
  [in13] -> M234/5(CT3)
  [in16] -> M234/6(MR3)
  [in17] -> M234/7(T3)
  [in18] -> M234/8(EB3)
  M234/1(LL1) -> Eval233/1(In1)
  M234/2(LL3) -> Eval233/2(In3)
  Eval233/1(Out1) -> To Workspace233/1
  [in1] -> M235/1(CT1)
  [in4] -> M235/2(MR1)
  [in5] -> M235/3(T1)
  [in6] -> M235/4(EB1)
  [in13] -> M235/5(CT3)
  [in16] -> M235/6(MR3)
  [in17] -> M235/7(T3)
  [in18] -> M235/8(EB3)
  M235/1(LL1) -> Eval234/1(In1)
  M235/2(LL3) -> Eval234/2(In3)
  Eval234/1(Out1) -> To Workspace234/1
  [in1] -> M236/1(CT1)
  [in4] -> M236/2(MR1)
  [in5] -> M236/3(T1)
  [in6] -> M236/4(EB1)
  [in13] -> M236/5(CT3)
  [in16] -> M236/6(MR3)
  [in17] -> M236/7(T3)
  [in18] -> M236/8(EB3)
  M236/1(LL1) -> Eval235/1(In1)
  M236/2(LL3) -> Eval235/2(In3)
  Eval235/1(Out1) -> To Workspace235/1
  [in1] -> M237/1(CT1)
  [in4] -> M237/2(MR1)
  [in5] -> M237/3(T1)
  [in6] -> M237/4(EB1)
  [in13] -> M237/5(CT3)
  [in16] -> M237/6(MR3)
  [in17] -> M237/7(T3)
  [in18] -> M237/8(EB3)
  M237/1(LL1) -> Eval236/1(In1)
  M237/2(LL3) -> Eval236/2(In3)
  Eval236/1(Out1) -> To Workspace236/1
  [in1] -> M238/1(CT1)
  [in4] -> M238/2(MR1)
  [in5] -> M238/3(T1)
  [in6] -> M238/4(EB1)
  [in13] -> M238/5(CT3)
  [in16] -> M238/6(MR3)
  [in17] -> M238/7(T3)
  [in18] -> M238/8(EB3)
  M238/1(LL1) -> Eval237/1(In1)
  M238/2(LL3) -> Eval237/2(In3)
  Eval237/1(Out1) -> To Workspace237/1
  [in1] -> M239/1(CT1)
  [in4] -> M239/2(MR1)
  [in5] -> M239/3(T1)
  [in6] -> M239/4(EB1)
  [in13] -> M239/5(CT3)
  [in16] -> M239/6(MR3)
  [in17] -> M239/7(T3)
  [in18] -> M239/8(EB3)
  M239/1(LL1) -> Eval238/1(In1)
  M239/2(LL3) -> Eval238/2(In3)
  Eval238/1(Out1) -> To Workspace238/1
  [in1] -> M240/1(CT1)
  [in4] -> M240/2(MR1)
  [in5] -> M240/3(T1)
  [in6] -> M240/4(EB1)
  [in13] -> M240/5(CT3)
  [in16] -> M240/6(MR3)
  [in17] -> M240/7(T3)
  [in18] -> M240/8(EB3)
  M240/1(LL1) -> Eval239/1(In1)
  M240/2(LL3) -> Eval239/2(In3)
  Eval239/1(Out1) -> To Workspace239/1
  [in1] -> M241/1(CT1)
  [in4] -> M241/2(MR1)
  [in5] -> M241/3(T1)
  [in6] -> M241/4(EB1)
  [in13] -> M241/5(CT3)
  [in16] -> M241/6(MR3)
  [in17] -> M241/7(T3)
  [in18] -> M241/8(EB3)
  M241/1(LL1) -> Eval240/1(In1)
  M241/2(LL3) -> Eval240/2(In3)
  Eval240/1(Out1) -> To Workspace240/1
  [in1] -> M242/1(CT1)
  [in4] -> M242/2(MR1)
  [in5] -> M242/3(T1)
  [in6] -> M242/4(EB1)
  [in13] -> M242/5(CT3)
  [in16] -> M242/6(MR3)
  [in17] -> M242/7(T3)
  [in18] -> M242/8(EB3)
  M242/1(LL1) -> Eval241/1(In1)
  M242/2(LL3) -> Eval241/2(In3)
  Eval241/1(Out1) -> To Workspace241/1
  [in1] -> M243/1(CT1)
  [in4] -> M243/2(MR1)
  [in5] -> M243/3(T1)
  [in6] -> M243/4(EB1)
  [in13] -> M243/5(CT3)
  [in16] -> M243/6(MR3)
  [in17] -> M243/7(T3)
  [in18] -> M243/8(EB3)
  M243/1(LL1) -> Eval242/1(In1)
  M243/2(LL3) -> Eval242/2(In3)
  Eval242/1(Out1) -> To Workspace242/1
  [in1] -> M244/1(CT1)
  [in4] -> M244/2(MR1)
  [in5] -> M244/3(T1)
  [in6] -> M244/4(EB1)
  [in13] -> M244/5(CT3)
  [in16] -> M244/6(MR3)
  [in17] -> M244/7(T3)
  [in18] -> M244/8(EB3)
  M244/1(LL1) -> Eval243/1(In1)
  M244/2(LL3) -> Eval243/2(In3)
  Eval243/1(Out1) -> To Workspace243/1
  [in1] -> M245/1(CT1)
  [in4] -> M245/2(MR1)
  [in5] -> M245/3(T1)
  [in6] -> M245/4(EB1)
  [in13] -> M245/5(CT3)
  [in16] -> M245/6(MR3)
  [in17] -> M245/7(T3)
  [in18] -> M245/8(EB3)
  M245/1(LL1) -> Eval244/1(In1)
  M245/2(LL3) -> Eval244/2(In3)
  Eval244/1(Out1) -> To Workspace244/1
  [in1] -> M246/1(CT1)
  [in4] -> M246/2(MR1)
  [in5] -> M246/3(T1)
  [in6] -> M246/4(EB1)
  [in13] -> M246/5(CT3)
  [in16] -> M246/6(MR3)
  [in17] -> M246/7(T3)
  [in18] -> M246/8(EB3)
  M246/1(LL1) -> Eval245/1(In1)
  M246/2(LL3) -> Eval245/2(In3)
  Eval245/1(Out1) -> To Workspace245/1
  Inputs/1(CT1) -> dtc_CT1/1
  dtc_CT1/1 -> CPSUT/1(CT1), [in1]
  Inputs/2(MR1) -> dtc_MR1/1
  dtc_MR1/1 -> CPSUT/2(MR1), [in4]
  Inputs/3(T1) -> dtc_T1/1
  dtc_T1/1 -> CPSUT/3(T1), [in5]
  Inputs/4(EB1) -> dtc_EB1/1
  dtc_EB1/1 -> CPSUT/4(EB1), [in6]
  Inputs/5(CT3) -> dtc_CT3/1
  dtc_CT3/1 -> CPSUT/5(CT3), [in13]
  Inputs/6(MR3) -> dtc_MR3/1
  dtc_MR3/1 -> CPSUT/6(MR3), [in16]
  Inputs/7(T3) -> dtc_T3/1
  dtc_T3/1 -> CPSUT/7(T3), [in17]
  Inputs/8(EB3) -> dtc_EB3/1
  dtc_EB3/1 -> CPSUT/8(EB3), [in18]

== system c00002M_harness/CPSUT ==
  note: VALUES
      | ---------------------------------
      | ControlType = 1 | 2 | 3
      | FillTank = 0 | 1
      | EmptyTank = 0 | 1
      | ManualReference between 0 and 1
      | Tempreature between 0 and 100
      | EmergencyButton = 0 | 1
      | LiquidLevel between 0 and 1 (hmax)
  note: Inputs For Tank2
  note: NAMES
      | --------------------------------------------
      | CT1 = ControlType Tank 1
      | F1 = Fill Tank 1
      | E1 = Empty Tank 1
      | MR1 = Manual Reference Tank1
      | T1 = Temperature Tank 1
      | EB1 = Emergency Button Tank 1
      | LL1 = Liquid Level 1
  note: Inputs For Tank3
  note: Inputs For Tank1
  CT1 : Inport
  MR1 : Inport  Port=2
  T1 : Inport  Port=3
  EB1 : Inport  Port=4
  CT3 : Inport  Port=5
  MR3 : Inport  Port=6
  T3 : Inport  Port=7
  EB3 : Inport  Port=8
  Tank1 : Subsystem
  Tank3 : Subsystem
  LL1 : Outport
  LL3 : Outport  Port=2
  wires:
  EB1/1 -> Tank1/4(EB1)
  Tank3/1(LL3) -> LL3/1
  MR3/1 -> Tank3/2(MR3)
  MR1/1 -> Tank1/2(MR1)
  T1/1 -> Tank1/3(T1)
  Tank1/1(LL1) -> LL1/1
  CT3/1 -> Tank3/1(CT3)
  EB3/1 -> Tank3/4(EB3)
  T3/1 -> Tank3/3(T3)
  CT1/1 -> Tank1/1(CT1)

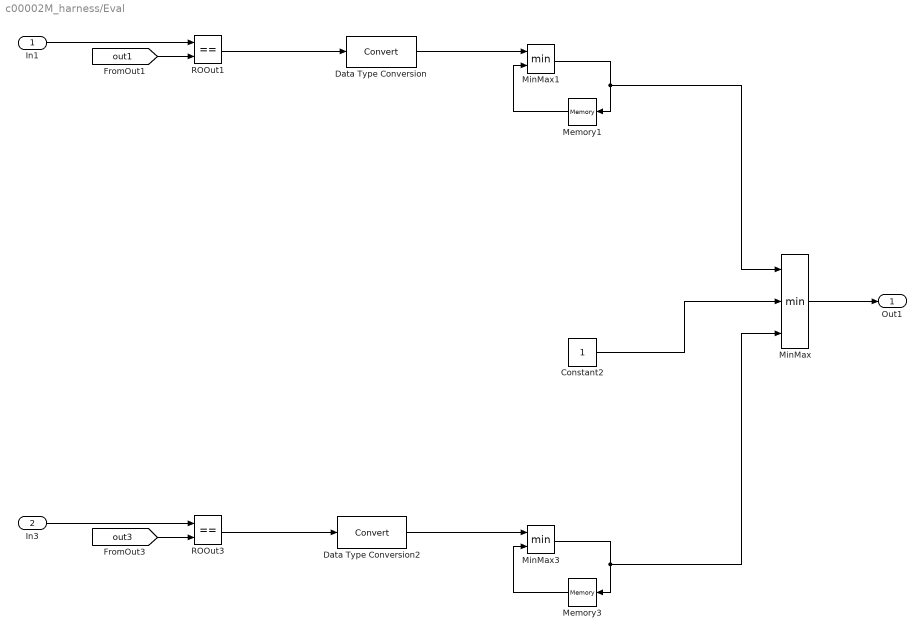
== system c00002M_harness/Eval ==
  In1 : Inport
  In3 : Inport  Port=2
  Constant2 : Constant
  Data Type Conversion : DataTypeConversion
  Data Type Conversion2 : DataTypeConversion
  Memory1 : Memory  InitialCondition=1
  Memory3 : Memory  InitialCondition=1
  MinMax : MinMax  Inputs=3
  MinMax1 : MinMax  Inputs=2
  MinMax3 : MinMax  Inputs=2
  ROOut1 : RelationalOperator  Operator===  OutDataTypeStr=boolean  RndMeth=Simplest
  ROOut3 : RelationalOperator  Operator===  OutDataTypeStr=boolean  RndMeth=Simplest
  Out1 : Outport
  wires:
  MinMax/1 -> Out1/1
  [out3] -> ROOut3/2
  In3/1 -> ROOut3/1
  [out1] -> ROOut1/2
  In1/1 -> ROOut1/1
  Memory1/1 -> MinMax1/2
  MinMax3/1 -> MinMax/3, Memory3/1
  ROOut3/1 -> Data Type Conversion2/1
  Memory3/1 -> MinMax3/2
  ROOut1/1 -> Data Type Conversion/1
  MinMax1/1 -> MinMax/1, Memory1/1
  Data Type Conversion/1 -> MinMax1/1
  Data Type Conversion2/1 -> MinMax3/1
  Constant2/1 -> MinMax/2

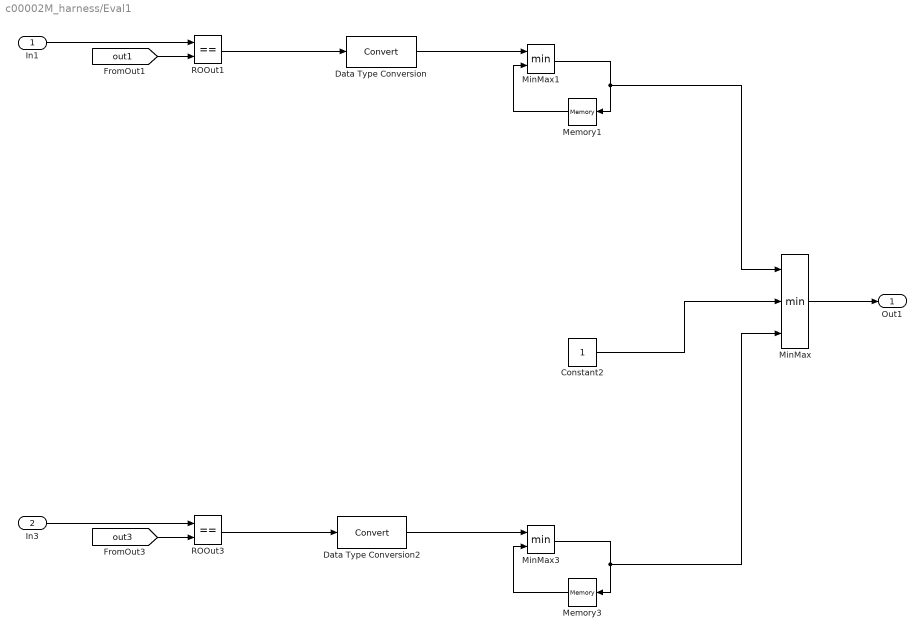
== system c00002M_harness/Eval1 ==
  In1 : Inport
  In3 : Inport  Port=2
  Constant2 : Constant
  Data Type Conversion : DataTypeConversion
  Data Type Conversion2 : DataTypeConversion
  Memory1 : Memory  InitialCondition=1
  Memory3 : Memory  InitialCondition=1
  MinMax : MinMax  Inputs=3
  MinMax1 : MinMax  Inputs=2
  MinMax3 : MinMax  Inputs=2
  ROOut1 : RelationalOperator  Operator===  OutDataTypeStr=boolean  RndMeth=Simplest
  ROOut3 : RelationalOperator  Operator===  OutDataTypeStr=boolean  RndMeth=Simplest
  Out1 : Outport
  wires:
  Data Type Conversion2/1 -> MinMax3/1
  Data Type Conversion/1 -> MinMax1/1
  MinMax1/1 -> Memory1/1, MinMax/1
  ROOut1/1 -> Data Type Conversion/1
  Memory3/1 -> MinMax3/2
  ROOut3/1 -> Data Type Conversion2/1
  MinMax3/1 -> Memory3/1, MinMax/3
  Memory1/1 -> MinMax1/2
  In1/1 -> ROOut1/1
  [out1] -> ROOut1/2
  In3/1 -> ROOut3/1
  [out3] -> ROOut3/2
  MinMax/1 -> Out1/1
  Constant2/1 -> MinMax/2

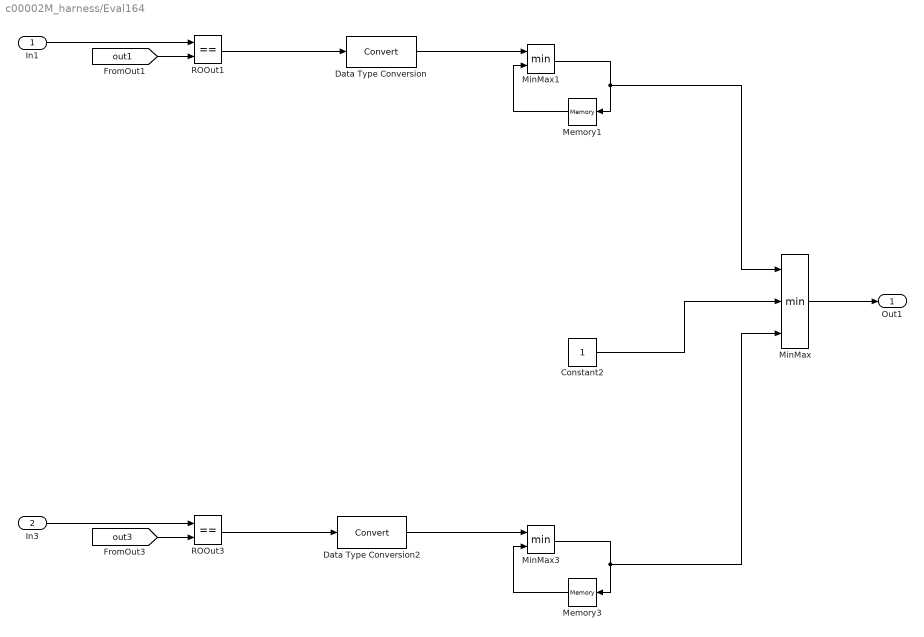
== system c00002M_harness/Eval164 ==
  In1 : Inport
  In3 : Inport  Port=2
  Constant2 : Constant
  Data Type Conversion : DataTypeConversion
  Data Type Conversion2 : DataTypeConversion
  Memory1 : Memory  InitialCondition=1
  Memory3 : Memory  InitialCondition=1
  MinMax : MinMax  Inputs=3
  MinMax1 : MinMax  Inputs=2
  MinMax3 : MinMax  Inputs=2
  ROOut1 : RelationalOperator  Operator===  OutDataTypeStr=boolean  RndMeth=Simplest
  ROOut3 : RelationalOperator  Operator===  OutDataTypeStr=boolean  RndMeth=Simplest
  Out1 : Outport
  wires:
  Data Type Conversion2/1 -> MinMax3/1
  Data Type Conversion/1 -> MinMax1/1
  MinMax1/1 -> Memory1/1, MinMax/1
  ROOut1/1 -> Data Type Conversion/1
  Memory3/1 -> MinMax3/2
  ROOut3/1 -> Data Type Conversion2/1
  MinMax3/1 -> Memory3/1, MinMax/3
  Memory1/1 -> MinMax1/2
  In1/1 -> ROOut1/1
  [out1] -> ROOut1/2
  In3/1 -> ROOut3/1
  [out3] -> ROOut3/2
  MinMax/1 -> Out1/1
  Constant2/1 -> MinMax/2

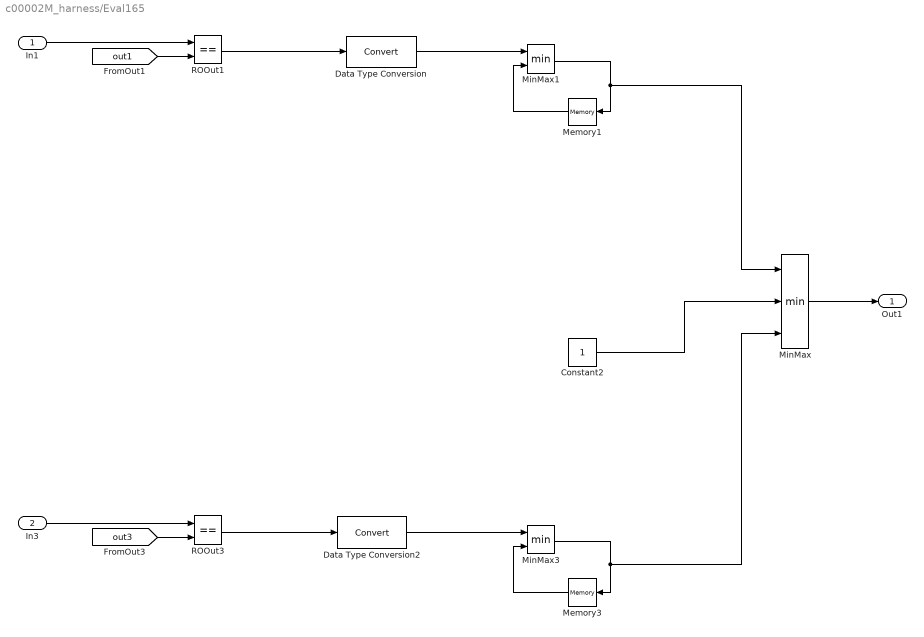
== system c00002M_harness/Eval165 ==
  In1 : Inport
  In3 : Inport  Port=2
  Constant2 : Constant
  Data Type Conversion : DataTypeConversion
  Data Type Conversion2 : DataTypeConversion
  Memory1 : Memory  InitialCondition=1
  Memory3 : Memory  InitialCondition=1
  MinMax : MinMax  Inputs=3
  MinMax1 : MinMax  Inputs=2
  MinMax3 : MinMax  Inputs=2
  ROOut1 : RelationalOperator  Operator===  OutDataTypeStr=boolean  RndMeth=Simplest
  ROOut3 : RelationalOperator  Operator===  OutDataTypeStr=boolean  RndMeth=Simplest
  Out1 : Outport
  wires:
  Data Type Conversion2/1 -> MinMax3/1
  Data Type Conversion/1 -> MinMax1/1
  MinMax1/1 -> Memory1/1, MinMax/1
  ROOut1/1 -> Data Type Conversion/1
  Memory3/1 -> MinMax3/2
  ROOut3/1 -> Data Type Conversion2/1
  MinMax3/1 -> Memory3/1, MinMax/3
  Memory1/1 -> MinMax1/2
  In1/1 -> ROOut1/1
  [out1] -> ROOut1/2
  In3/1 -> ROOut3/1
  [out3] -> ROOut3/2
  MinMax/1 -> Out1/1
  Constant2/1 -> MinMax/2

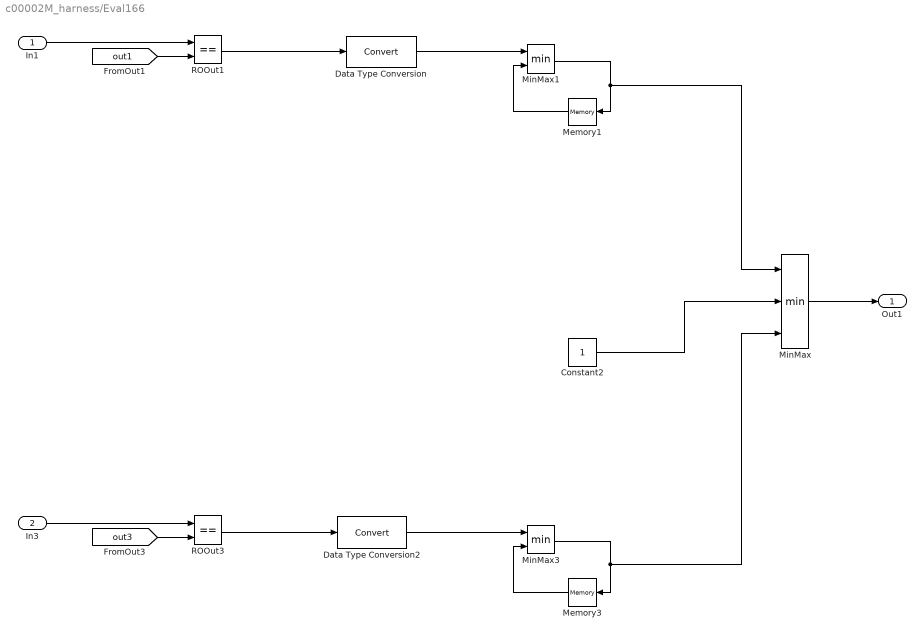
== system c00002M_harness/Eval166 ==
  In1 : Inport
  In3 : Inport  Port=2
  Constant2 : Constant
  Data Type Conversion : DataTypeConversion
  Data Type Conversion2 : DataTypeConversion
  Memory1 : Memory  InitialCondition=1
  Memory3 : Memory  InitialCondition=1
  MinMax : MinMax  Inputs=3
  MinMax1 : MinMax  Inputs=2
  MinMax3 : MinMax  Inputs=2
  ROOut1 : RelationalOperator  Operator===  OutDataTypeStr=boolean  RndMeth=Simplest
  ROOut3 : RelationalOperator  Operator===  OutDataTypeStr=boolean  RndMeth=Simplest
  Out1 : Outport
  wires:
  Data Type Conversion2/1 -> MinMax3/1
  Data Type Conversion/1 -> MinMax1/1
  MinMax1/1 -> Memory1/1, MinMax/1
  ROOut1/1 -> Data Type Conversion/1
  Memory3/1 -> MinMax3/2
  ROOut3/1 -> Data Type Conversion2/1
  MinMax3/1 -> Memory3/1, MinMax/3
  Memory1/1 -> MinMax1/2
  In1/1 -> ROOut1/1
  [out1] -> ROOut1/2
  In3/1 -> ROOut3/1
  [out3] -> ROOut3/2
  MinMax/1 -> Out1/1
  Constant2/1 -> MinMax/2

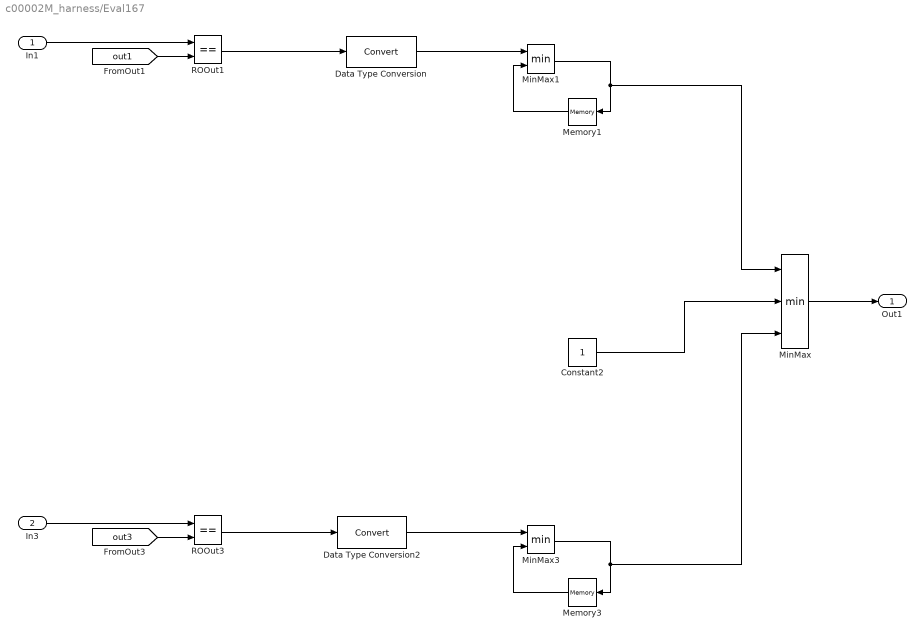
== system c00002M_harness/Eval167 ==
  In1 : Inport
  In3 : Inport  Port=2
  Constant2 : Constant
  Data Type Conversion : DataTypeConversion
  Data Type Conversion2 : DataTypeConversion
  Memory1 : Memory  InitialCondition=1
  Memory3 : Memory  InitialCondition=1
  MinMax : MinMax  Inputs=3
  MinMax1 : MinMax  Inputs=2
  MinMax3 : MinMax  Inputs=2
  ROOut1 : RelationalOperator  Operator===  OutDataTypeStr=boolean  RndMeth=Simplest
  ROOut3 : RelationalOperator  Operator===  OutDataTypeStr=boolean  RndMeth=Simplest
  Out1 : Outport
  wires:
  Data Type Conversion2/1 -> MinMax3/1
  Data Type Conversion/1 -> MinMax1/1
  MinMax1/1 -> Memory1/1, MinMax/1
  ROOut1/1 -> Data Type Conversion/1
  Memory3/1 -> MinMax3/2
  ROOut3/1 -> Data Type Conversion2/1
  MinMax3/1 -> Memory3/1, MinMax/3
  Memory1/1 -> MinMax1/2
  In1/1 -> ROOut1/1
  [out1] -> ROOut1/2
  In3/1 -> ROOut3/1
  [out3] -> ROOut3/2
  MinMax/1 -> Out1/1
  Constant2/1 -> MinMax/2

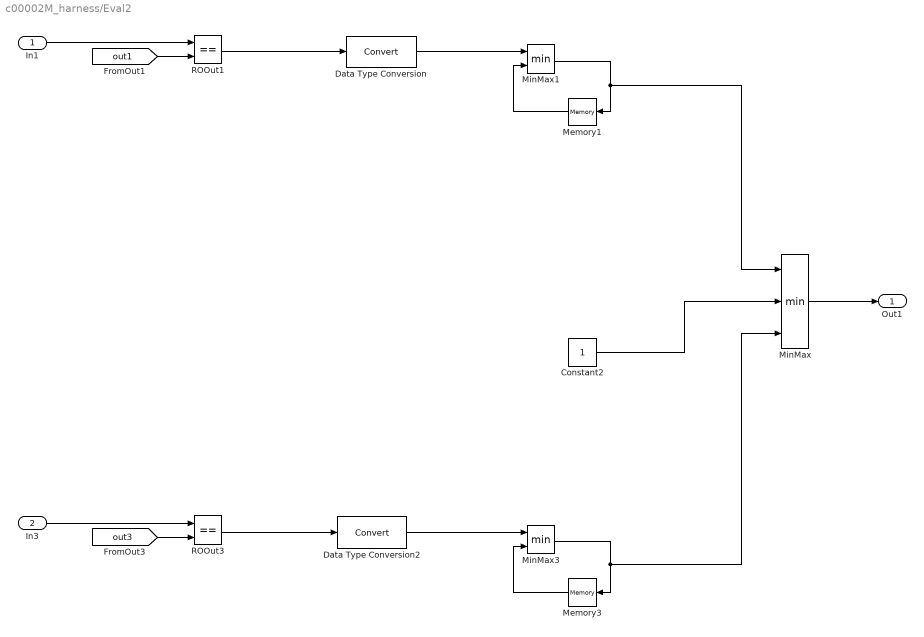
== system c00002M_harness/Eval2 ==
  In1 : Inport
  In3 : Inport  Port=2
  Constant2 : Constant
  Data Type Conversion : DataTypeConversion
  Data Type Conversion2 : DataTypeConversion
  Memory1 : Memory  InitialCondition=1
  Memory3 : Memory  InitialCondition=1
  MinMax : MinMax  Inputs=3
  MinMax1 : MinMax  Inputs=2
  MinMax3 : MinMax  Inputs=2
  ROOut1 : RelationalOperator  Operator===  OutDataTypeStr=boolean  RndMeth=Simplest
  ROOut3 : RelationalOperator  Operator===  OutDataTypeStr=boolean  RndMeth=Simplest
  Out1 : Outport
  wires:
  Data Type Conversion2/1 -> MinMax3/1
  Data Type Conversion/1 -> MinMax1/1
  MinMax1/1 -> Memory1/1, MinMax/1
  ROOut1/1 -> Data Type Conversion/1
  Memory3/1 -> MinMax3/2
  ROOut3/1 -> Data Type Conversion2/1
  MinMax3/1 -> Memory3/1, MinMax/3
  Memory1/1 -> MinMax1/2
  In1/1 -> ROOut1/1
  [out1] -> ROOut1/2
  In3/1 -> ROOut3/1
  [out3] -> ROOut3/2
  MinMax/1 -> Out1/1
  Constant2/1 -> MinMax/2

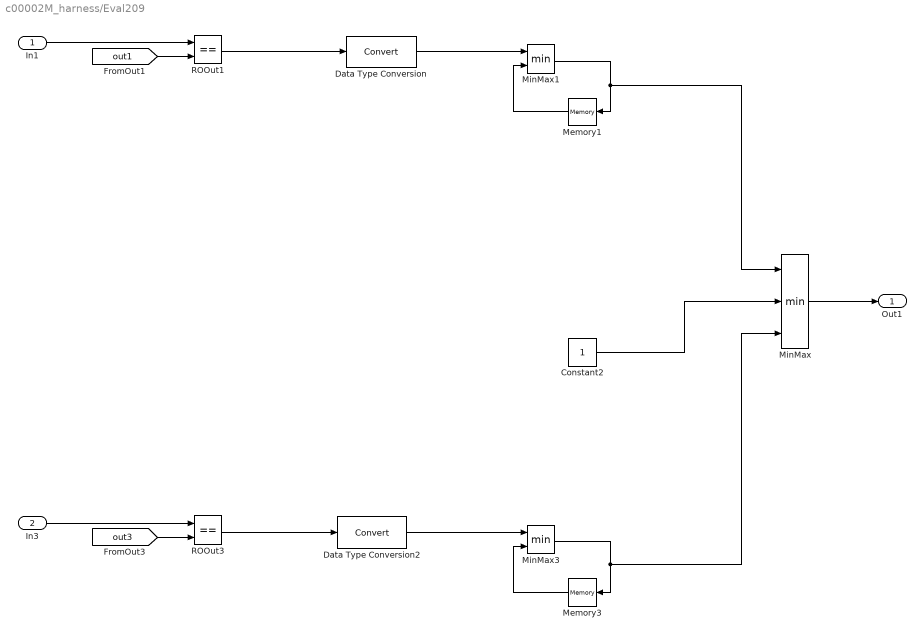
== system c00002M_harness/Eval209 ==
  In1 : Inport
  In3 : Inport  Port=2
  Constant2 : Constant
  Data Type Conversion : DataTypeConversion
  Data Type Conversion2 : DataTypeConversion
  Memory1 : Memory  InitialCondition=1
  Memory3 : Memory  InitialCondition=1
  MinMax : MinMax  Inputs=3
  MinMax1 : MinMax  Inputs=2
  MinMax3 : MinMax  Inputs=2
  ROOut1 : RelationalOperator  Operator===  OutDataTypeStr=boolean  RndMeth=Simplest
  ROOut3 : RelationalOperator  Operator===  OutDataTypeStr=boolean  RndMeth=Simplest
  Out1 : Outport
  wires:
  Data Type Conversion2/1 -> MinMax3/1
  Data Type Conversion/1 -> MinMax1/1
  MinMax1/1 -> Memory1/1, MinMax/1
  ROOut1/1 -> Data Type Conversion/1
  Memory3/1 -> MinMax3/2
  ROOut3/1 -> Data Type Conversion2/1
  MinMax3/1 -> Memory3/1, MinMax/3
  Memory1/1 -> MinMax1/2
  In1/1 -> ROOut1/1
  [out1] -> ROOut1/2
  In3/1 -> ROOut3/1
  [out3] -> ROOut3/2
  MinMax/1 -> Out1/1
  Constant2/1 -> MinMax/2

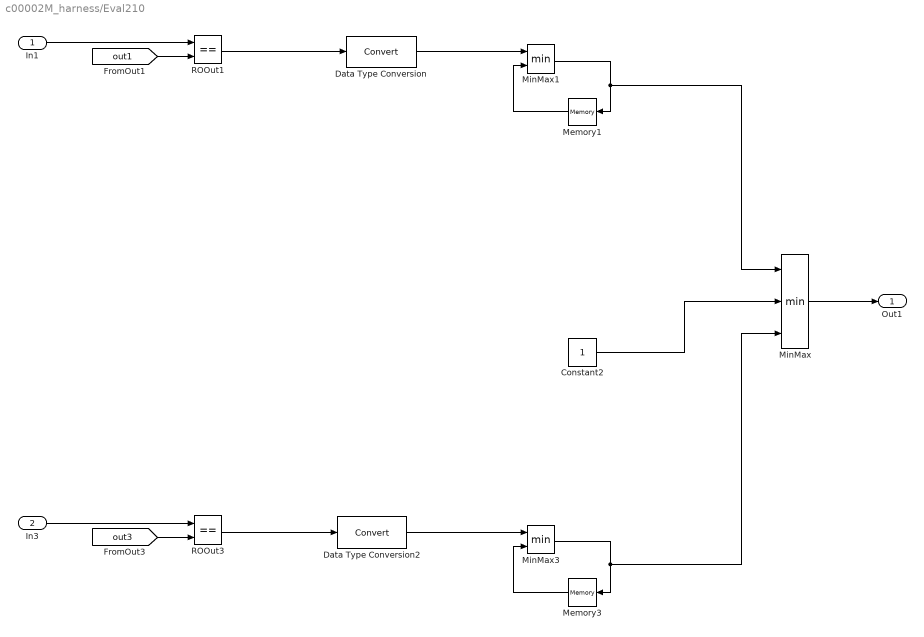
== system c00002M_harness/Eval210 ==
  In1 : Inport
  In3 : Inport  Port=2
  Constant2 : Constant
  Data Type Conversion : DataTypeConversion
  Data Type Conversion2 : DataTypeConversion
  Memory1 : Memory  InitialCondition=1
  Memory3 : Memory  InitialCondition=1
  MinMax : MinMax  Inputs=3
  MinMax1 : MinMax  Inputs=2
  MinMax3 : MinMax  Inputs=2
  ROOut1 : RelationalOperator  Operator===  OutDataTypeStr=boolean  RndMeth=Simplest
  ROOut3 : RelationalOperator  Operator===  OutDataTypeStr=boolean  RndMeth=Simplest
  Out1 : Outport
  wires:
  Data Type Conversion2/1 -> MinMax3/1
  Data Type Conversion/1 -> MinMax1/1
  MinMax1/1 -> Memory1/1, MinMax/1
  ROOut1/1 -> Data Type Conversion/1
  Memory3/1 -> MinMax3/2
  ROOut3/1 -> Data Type Conversion2/1
  MinMax3/1 -> Memory3/1, MinMax/3
  Memory1/1 -> MinMax1/2
  In1/1 -> ROOut1/1
  [out1] -> ROOut1/2
  In3/1 -> ROOut3/1
  [out3] -> ROOut3/2
  MinMax/1 -> Out1/1
  Constant2/1 -> MinMax/2

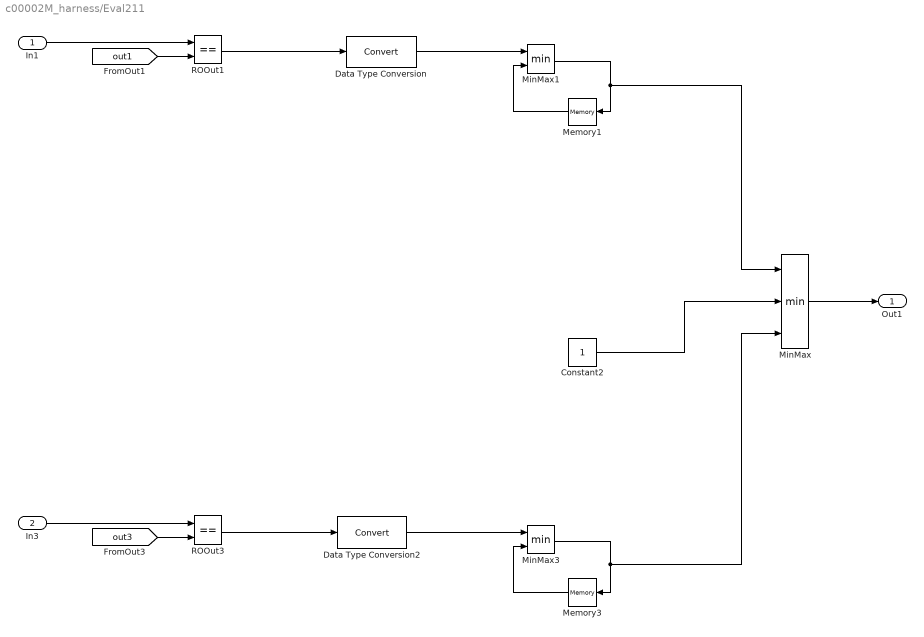
== system c00002M_harness/Eval211 ==
  In1 : Inport
  In3 : Inport  Port=2
  Constant2 : Constant
  Data Type Conversion : DataTypeConversion
  Data Type Conversion2 : DataTypeConversion
  Memory1 : Memory  InitialCondition=1
  Memory3 : Memory  InitialCondition=1
  MinMax : MinMax  Inputs=3
  MinMax1 : MinMax  Inputs=2
  MinMax3 : MinMax  Inputs=2
  ROOut1 : RelationalOperator  Operator===  OutDataTypeStr=boolean  RndMeth=Simplest
  ROOut3 : RelationalOperator  Operator===  OutDataTypeStr=boolean  RndMeth=Simplest
  Out1 : Outport
  wires:
  Data Type Conversion2/1 -> MinMax3/1
  Data Type Conversion/1 -> MinMax1/1
  MinMax1/1 -> Memory1/1, MinMax/1
  ROOut1/1 -> Data Type Conversion/1
  Memory3/1 -> MinMax3/2
  ROOut3/1 -> Data Type Conversion2/1
  MinMax3/1 -> Memory3/1, MinMax/3
  Memory1/1 -> MinMax1/2
  In1/1 -> ROOut1/1
  [out1] -> ROOut1/2
  In3/1 -> ROOut3/1
  [out3] -> ROOut3/2
  MinMax/1 -> Out1/1
  Constant2/1 -> MinMax/2

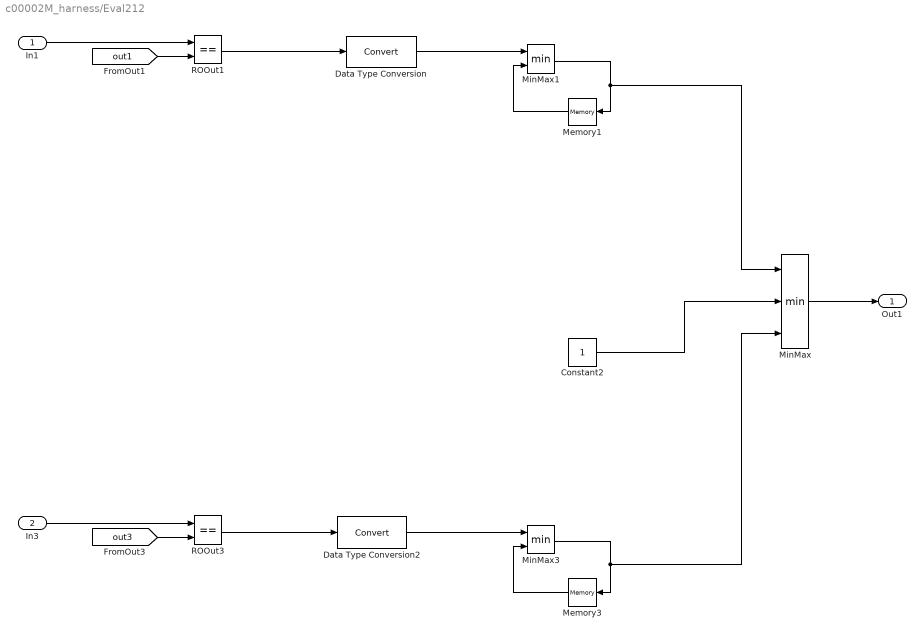
== system c00002M_harness/Eval212 ==
  In1 : Inport
  In3 : Inport  Port=2
  Constant2 : Constant
  Data Type Conversion : DataTypeConversion
  Data Type Conversion2 : DataTypeConversion
  Memory1 : Memory  InitialCondition=1
  Memory3 : Memory  InitialCondition=1
  MinMax : MinMax  Inputs=3
  MinMax1 : MinMax  Inputs=2
  MinMax3 : MinMax  Inputs=2
  ROOut1 : RelationalOperator  Operator===  OutDataTypeStr=boolean  RndMeth=Simplest
  ROOut3 : RelationalOperator  Operator===  OutDataTypeStr=boolean  RndMeth=Simplest
  Out1 : Outport
  wires:
  Data Type Conversion2/1 -> MinMax3/1
  Data Type Conversion/1 -> MinMax1/1
  MinMax1/1 -> Memory1/1, MinMax/1
  ROOut1/1 -> Data Type Conversion/1
  Memory3/1 -> MinMax3/2
  ROOut3/1 -> Data Type Conversion2/1
  MinMax3/1 -> Memory3/1, MinMax/3
  Memory1/1 -> MinMax1/2
  In1/1 -> ROOut1/1
  [out1] -> ROOut1/2
  In3/1 -> ROOut3/1
  [out3] -> ROOut3/2
  MinMax/1 -> Out1/1
  Constant2/1 -> MinMax/2

== system c00002M_harness/Eval213 ==
  In1 : Inport
  In3 : Inport  Port=2
  Constant2 : Constant
  Data Type Conversion : DataTypeConversion
  Data Type Conversion2 : DataTypeConversion
  Memory1 : Memory  InitialCondition=1
  Memory3 : Memory  InitialCondition=1
  MinMax : MinMax  Inputs=3
  MinMax1 : MinMax  Inputs=2
  MinMax3 : MinMax  Inputs=2
  ROOut1 : RelationalOperator  Operator===  OutDataTypeStr=boolean  RndMeth=Simplest
  ROOut3 : RelationalOperator  Operator===  OutDataTypeStr=boolean  RndMeth=Simplest
  Out1 : Outport
  wires:
  Data Type Conversion2/1 -> MinMax3/1
  Data Type Conversion/1 -> MinMax1/1
  MinMax1/1 -> Memory1/1, MinMax/1
  ROOut1/1 -> Data Type Conversion/1
  Memory3/1 -> MinMax3/2
  ROOut3/1 -> Data Type Conversion2/1
  MinMax3/1 -> Memory3/1, MinMax/3
  Memory1/1 -> MinMax1/2
  In1/1 -> ROOut1/1
  [out1] -> ROOut1/2
  In3/1 -> ROOut3/1
  [out3] -> ROOut3/2
  MinMax/1 -> Out1/1
  Constant2/1 -> MinMax/2

== system c00002M_harness/Eval214 ==
  In1 : Inport
  In3 : Inport  Port=2
  Constant2 : Constant
  Data Type Conversion : DataTypeConversion
  Data Type Conversion2 : DataTypeConversion
  Memory1 : Memory  InitialCondition=1
  Memory3 : Memory  InitialCondition=1
  MinMax : MinMax  Inputs=3
  MinMax1 : MinMax  Inputs=2
  MinMax3 : MinMax  Inputs=2
  ROOut1 : RelationalOperator  Operator===  OutDataTypeStr=boolean  RndMeth=Simplest
  ROOut3 : RelationalOperator  Operator===  OutDataTypeStr=boolean  RndMeth=Simplest
  Out1 : Outport
  wires:
  Data Type Conversion2/1 -> MinMax3/1
  Data Type Conversion/1 -> MinMax1/1
  MinMax1/1 -> Memory1/1, MinMax/1
  ROOut1/1 -> Data Type Conversion/1
  Memory3/1 -> MinMax3/2
  ROOut3/1 -> Data Type Conversion2/1
  MinMax3/1 -> Memory3/1, MinMax/3
  Memory1/1 -> MinMax1/2
  In1/1 -> ROOut1/1
  [out1] -> ROOut1/2
  In3/1 -> ROOut3/1
  [out3] -> ROOut3/2
  MinMax/1 -> Out1/1
  Constant2/1 -> MinMax/2

== system c00002M_harness/Eval215 ==
  In1 : Inport
  In3 : Inport  Port=2
  Constant2 : Constant
  Data Type Conversion : DataTypeConversion
  Data Type Conversion2 : DataTypeConversion
  Memory1 : Memory  InitialCondition=1
  Memory3 : Memory  InitialCondition=1
  MinMax : MinMax  Inputs=3
  MinMax1 : MinMax  Inputs=2
  MinMax3 : MinMax  Inputs=2
  ROOut1 : RelationalOperator  Operator===  OutDataTypeStr=boolean  RndMeth=Simplest
  ROOut3 : RelationalOperator  Operator===  OutDataTypeStr=boolean  RndMeth=Simplest
  Out1 : Outport
  wires:
  Data Type Conversion2/1 -> MinMax3/1
  Data Type Conversion/1 -> MinMax1/1
  MinMax1/1 -> Memory1/1, MinMax/1
  ROOut1/1 -> Data Type Conversion/1
  Memory3/1 -> MinMax3/2
  ROOut3/1 -> Data Type Conversion2/1
  MinMax3/1 -> Memory3/1, MinMax/3
  Memory1/1 -> MinMax1/2
  In1/1 -> ROOut1/1
  [out1] -> ROOut1/2
  In3/1 -> ROOut3/1
  [out3] -> ROOut3/2
  MinMax/1 -> Out1/1
  Constant2/1 -> MinMax/2

== system c00002M_harness/Eval216 ==
  In1 : Inport
  In3 : Inport  Port=2
  Constant2 : Constant
  Data Type Conversion : DataTypeConversion
  Data Type Conversion2 : DataTypeConversion
  Memory1 : Memory  InitialCondition=1
  Memory3 : Memory  InitialCondition=1
  MinMax : MinMax  Inputs=3
  MinMax1 : MinMax  Inputs=2
  MinMax3 : MinMax  Inputs=2
  ROOut1 : RelationalOperator  Operator===  OutDataTypeStr=boolean  RndMeth=Simplest
  ROOut3 : RelationalOperator  Operator===  OutDataTypeStr=boolean  RndMeth=Simplest
  Out1 : Outport
  wires:
  Data Type Conversion2/1 -> MinMax3/1
  Data Type Conversion/1 -> MinMax1/1
  MinMax1/1 -> Memory1/1, MinMax/1
  ROOut1/1 -> Data Type Conversion/1
  Memory3/1 -> MinMax3/2
  ROOut3/1 -> Data Type Conversion2/1
  MinMax3/1 -> Memory3/1, MinMax/3
  Memory1/1 -> MinMax1/2
  In1/1 -> ROOut1/1
  [out1] -> ROOut1/2
  In3/1 -> ROOut3/1
  [out3] -> ROOut3/2
  MinMax/1 -> Out1/1
  Constant2/1 -> MinMax/2

== system c00002M_harness/Eval217 ==
  In1 : Inport
  In3 : Inport  Port=2
  Constant2 : Constant
  Data Type Conversion : DataTypeConversion
  Data Type Conversion2 : DataTypeConversion
  Memory1 : Memory  InitialCondition=1
  Memory3 : Memory  InitialCondition=1
  MinMax : MinMax  Inputs=3
  MinMax1 : MinMax  Inputs=2
  MinMax3 : MinMax  Inputs=2
  ROOut1 : RelationalOperator  Operator===  OutDataTypeStr=boolean  RndMeth=Simplest
  ROOut3 : RelationalOperator  Operator===  OutDataTypeStr=boolean  RndMeth=Simplest
  Out1 : Outport
  wires:
  Data Type Conversion2/1 -> MinMax3/1
  Data Type Conversion/1 -> MinMax1/1
  MinMax1/1 -> Memory1/1, MinMax/1
  ROOut1/1 -> Data Type Conversion/1
  Memory3/1 -> MinMax3/2
  ROOut3/1 -> Data Type Conversion2/1
  MinMax3/1 -> Memory3/1, MinMax/3
  Memory1/1 -> MinMax1/2
  In1/1 -> ROOut1/1
  [out1] -> ROOut1/2
  In3/1 -> ROOut3/1
  [out3] -> ROOut3/2
  MinMax/1 -> Out1/1
  Constant2/1 -> MinMax/2

== system c00002M_harness/Eval218 ==
  In1 : Inport
  In3 : Inport  Port=2
  Constant2 : Constant
  Data Type Conversion : DataTypeConversion
  Data Type Conversion2 : DataTypeConversion
  Memory1 : Memory  InitialCondition=1
  Memory3 : Memory  InitialCondition=1
  MinMax : MinMax  Inputs=3
  MinMax1 : MinMax  Inputs=2
  MinMax3 : MinMax  Inputs=2
  ROOut1 : RelationalOperator  Operator===  OutDataTypeStr=boolean  RndMeth=Simplest
  ROOut3 : RelationalOperator  Operator===  OutDataTypeStr=boolean  RndMeth=Simplest
  Out1 : Outport
  wires:
  Data Type Conversion2/1 -> MinMax3/1
  Data Type Conversion/1 -> MinMax1/1
  MinMax1/1 -> Memory1/1, MinMax/1
  ROOut1/1 -> Data Type Conversion/1
  Memory3/1 -> MinMax3/2
  ROOut3/1 -> Data Type Conversion2/1
  MinMax3/1 -> Memory3/1, MinMax/3
  Memory1/1 -> MinMax1/2
  In1/1 -> ROOut1/1
  [out1] -> ROOut1/2
  In3/1 -> ROOut3/1
  [out3] -> ROOut3/2
  MinMax/1 -> Out1/1
  Constant2/1 -> MinMax/2

== system c00002M_harness/Eval219 ==
  In1 : Inport
  In3 : Inport  Port=2
  Constant2 : Constant
  Data Type Conversion : DataTypeConversion
  Data Type Conversion2 : DataTypeConversion
  Memory1 : Memory  InitialCondition=1
  Memory3 : Memory  InitialCondition=1
  MinMax : MinMax  Inputs=3
  MinMax1 : MinMax  Inputs=2
  MinMax3 : MinMax  Inputs=2
  ROOut1 : RelationalOperator  Operator===  OutDataTypeStr=boolean  RndMeth=Simplest
  ROOut3 : RelationalOperator  Operator===  OutDataTypeStr=boolean  RndMeth=Simplest
  Out1 : Outport
  wires:
  Data Type Conversion2/1 -> MinMax3/1
  Data Type Conversion/1 -> MinMax1/1
  MinMax1/1 -> Memory1/1, MinMax/1
  ROOut1/1 -> Data Type Conversion/1
  Memory3/1 -> MinMax3/2
  ROOut3/1 -> Data Type Conversion2/1
  MinMax3/1 -> Memory3/1, MinMax/3
  Memory1/1 -> MinMax1/2
  In1/1 -> ROOut1/1
  [out1] -> ROOut1/2
  In3/1 -> ROOut3/1
  [out3] -> ROOut3/2
  MinMax/1 -> Out1/1
  Constant2/1 -> MinMax/2

== system c00002M_harness/Eval220 ==
  In1 : Inport
  In3 : Inport  Port=2
  Constant2 : Constant
  Data Type Conversion : DataTypeConversion
  Data Type Conversion2 : DataTypeConversion
  Memory1 : Memory  InitialCondition=1
  Memory3 : Memory  InitialCondition=1
  MinMax : MinMax  Inputs=3
  MinMax1 : MinMax  Inputs=2
  MinMax3 : MinMax  Inputs=2
  ROOut1 : RelationalOperator  Operator===  OutDataTypeStr=boolean  RndMeth=Simplest
  ROOut3 : RelationalOperator  Operator===  OutDataTypeStr=boolean  RndMeth=Simplest
  Out1 : Outport
  wires:
  Data Type Conversion2/1 -> MinMax3/1
  Data Type Conversion/1 -> MinMax1/1
  MinMax1/1 -> Memory1/1, MinMax/1
  ROOut1/1 -> Data Type Conversion/1
  Memory3/1 -> MinMax3/2
  ROOut3/1 -> Data Type Conversion2/1
  MinMax3/1 -> Memory3/1, MinMax/3
  Memory1/1 -> MinMax1/2
  In1/1 -> ROOut1/1
  [out1] -> ROOut1/2
  In3/1 -> ROOut3/1
  [out3] -> ROOut3/2
  MinMax/1 -> Out1/1
  Constant2/1 -> MinMax/2

== system c00002M_harness/Eval221 ==
  In1 : Inport
  In3 : Inport  Port=2
  Constant2 : Constant
  Data Type Conversion : DataTypeConversion
  Data Type Conversion2 : DataTypeConversion
  Memory1 : Memory  InitialCondition=1
  Memory3 : Memory  InitialCondition=1
  MinMax : MinMax  Inputs=3
  MinMax1 : MinMax  Inputs=2
  MinMax3 : MinMax  Inputs=2
  ROOut1 : RelationalOperator  Operator===  OutDataTypeStr=boolean  RndMeth=Simplest
  ROOut3 : RelationalOperator  Operator===  OutDataTypeStr=boolean  RndMeth=Simplest
  Out1 : Outport
  wires:
  Data Type Conversion2/1 -> MinMax3/1
  Data Type Conversion/1 -> MinMax1/1
  MinMax1/1 -> Memory1/1, MinMax/1
  ROOut1/1 -> Data Type Conversion/1
  Memory3/1 -> MinMax3/2
  ROOut3/1 -> Data Type Conversion2/1
  MinMax3/1 -> Memory3/1, MinMax/3
  Memory1/1 -> MinMax1/2
  In1/1 -> ROOut1/1
  [out1] -> ROOut1/2
  In3/1 -> ROOut3/1
  [out3] -> ROOut3/2
  MinMax/1 -> Out1/1
  Constant2/1 -> MinMax/2
